simulink model "Wiper_Control_System"  (R2024a)
settings: Solver=VariableStepAuto  StartTime=0.0  StopTime=10.0  RelTol=1e-3
settings Model: Creator=VICTUS  LastModifiedBy=VICTUS

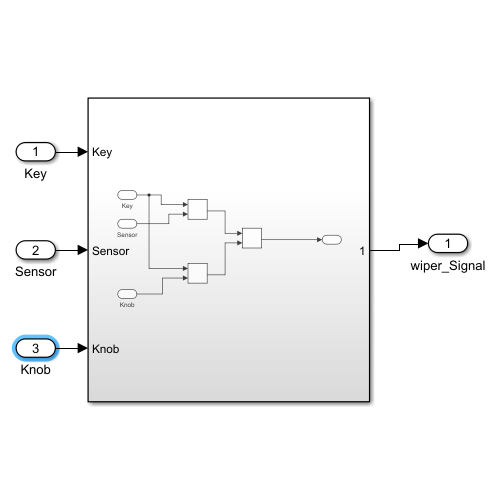
[thumbnail: Simulink's stored preview of the top-level diagram]
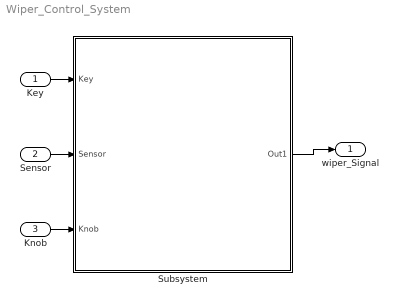
== system Wiper_Control_System ==
  Key : Inport
  Sensor : Inport  Port=2
  Knob : Inport  Port=3
  Subsystem : Subsystem
  wiper_Signal : Outport
  wires:
  Key/1 -> Subsystem/1(Key)
  Sensor/1 -> Subsystem/2(Sensor)
  Knob/1 -> Subsystem/3(Knob)
  Subsystem/1(Out1) -> wiper_Signal/1

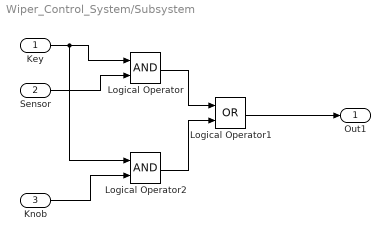
== system Wiper_Control_System/Subsystem ==
  Key : Inport
  Sensor : Inport  Port=2
  Knob : Inport  Port=3
  Logical Operator : Logic  AllPortsSameDT=off  OutDataTypeStr=boolean
  Logical Operator1 : Logic  Operator=OR  AllPortsSameDT=off  OutDataTypeStr=boolean
  Logical Operator2 : Logic  AllPortsSameDT=off  OutDataTypeStr=boolean
  Out1 : Outport
  wires:
  Logical Operator/1 -> Logical Operator1/1
  Knob/1 -> Logical Operator2/2
  Logical Operator2/1 -> Logical Operator1/2
  Key/1 -> Logical Operator2/1, Logical Operator/1
  Logical Operator1/1 -> Out1/1
  Sensor/1 -> Logical Operator/2
